simulink model "final_quadruped_060722_alphaobjfun"  (R2021a)
settings: Solver=ode15s  StartTime=0.0  StopTime=10  FixedStep=1e-3  RelTol=1e-5  EnableMultiTasking=on
values from neighbouring files (symbols this model uses):
  foot_x = 8    [bipedparameters.m]    (also in fcn.m; finalrobotParameters.m; finalrobotParameters_110522.m; finalrobotParameters_140522.m)
  foot_y = 6    [bipedparameters.m]    (also in fcn.m; finalrobotParameters.m; finalrobotParameters_110522.m; finalrobotParameters_140522.m)
  foot_z = 1    [bipedparameters.m]    (also in fcn.m; finalrobotParameters.m; finalrobotParameters_110522.m; finalrobotParameters_140522.m)
  height_plane = 0.025    [bipedparameters.m]    (also in finalrobotParameters.m; finalrobotParameters_110522.m; finalrobotParameters_140522.m; finalrobotParameters_240522.m)
  kd_ankle = 1000    [bipedparameters.m]    (also in finalrobotParameters_240522.m)
  kd_hip = 1000    [bipedparameters.m]    (also in finalrobotParameters_240522.m)
  kd_knee = 1000    [bipedparameters.m]    (also in finalrobotParameters_240522.m)
  ki_ankle = 1000    [bipedparameters.m]    (also in finalrobotParameters_240522.m)
  ki_hip = 1000    [bipedparameters.m]    (also in finalrobotParameters_240522.m)
  ki_knee = 2000    [bipedparameters.m]    (also in finalrobotParameters_240522.m)
  kp_ankle = 1000    [bipedparameters.m]    (also in finalrobotParameters_240522.m)
  kp_hip = 1000    [bipedparameters.m]    (also in finalrobotParameters_240522.m)
  kp_knee = 2000    [bipedparameters.m]    (also in finalrobotParameters_240522.m)
  lower_leg_length = 10    [bipedparameters.m]    (also in fcn.m; finalrobotParameters.m; finalrobotParameters_110522.m; finalrobotParameters_140522.m)
  plane_x = 25    [bipedparameters.m]    (also in finalrobotParameters.m; finalrobotParameters_110522.m; finalrobotParameters_140522.m; finalrobotParameters_240522.m)
  plane_y = 3    [bipedparameters.m]    (also in finalrobotParameters.m; finalrobotParameters_110522.m; finalrobotParameters_140522.m; finalrobotParameters_240522.m)
  torso_offset_x = -0.5    [bipedparameters.m]    (also in finalrobotParameters.m = 10; finalrobotParameters_110522.m = 10; finalrobotParameters_140522.m = 10; finalrobotParameters_240522.m = 10)
  torso_offset_z = -2    [bipedparameters.m]    (also in finalrobotParameters.m; finalrobotParameters_110522.m; finalrobotParameters_140522.m; finalrobotParameters_240522.m)
  torso_x = 5    [bipedparameters.m]    (also in fcn.m = 25; finalrobotParameters.m = 25; finalrobotParameters_110522.m = 25; finalrobotParameters_140522.m = 25)
  torso_y = 10    [bipedparameters.m]    (also in fcn.m = 16; finalrobotParameters.m = 16; finalrobotParameters_110522.m = 16; finalrobotParameters_140522.m = 16)
  torso_z = 8    [bipedparameters.m]    (also in fcn.m = 10; finalrobotParameters.m = 10; finalrobotParameters_110522.m = 10; finalrobotParameters_140522.m = 10)
  upper_leg_length = 10    [bipedparameters.m]    (also in fcn.m; finalrobotParameters.m; finalrobotParameters_110522.m; finalrobotParameters_140522.m)
undefined symbols (not defined in the file or in its folder): sigbuilder_block, X, Y, Z
libraries: nesl_utility x288, sm_lib x71, pid_lib x20, Contact_Forces_Lib x16, fl_lib x3
(part 6 of 9)

== system final_quadruped_060722_alphaobjfun/Model/Left Leg Front /Ankle  ==
  note: accelerationRFankle
  tddLF_ankle : Inport
  t2ddankle : Inport  Port=2
  Ankle : sm_lib/Joints/Revolute Joint  JointMode=Normal  SenseConstraintForce=off  SenseConstraintForceX=off  SenseConstraintForceY=off  SenseConstraintForceZ=off  SenseConstraintTorque=off  SenseConstraintTorqueX=off  SenseConstraintTorqueY=off  SenseConstraintTorqueZ=off  SenseTotalForce=off  SenseTotalForceX=off  SenseTotalForceY=off  SenseTotalForceZ=off  SenseTotalTorque=off  SenseTotalTorqueX=off  SenseTotalTorqueY=off  SenseTotalTorqueZ=off  CompositeWrenchDir=FollowerOnBase  CompositeWrenchFrame=BaseFrame  EquilibriumPosition=0  EquilibriumPositionUnits=deg  SpringStiffness=0  SpringStiffnessUnits=N*m/deg  DampingCoefficient=0  DampingCoefficientUnits=N*m/(deg/s)  TorqueActuationMode=InputTorque  MotionActuationMode=ComputedMotion  SensePosition=on  SenseVelocity=on  SenseAcceleration=on  SenseTorqueForce=off  SenseLowerLimitTorqueForce=off  SenseUpperLimitTorqueForce=off  LowerLimitSpecify=off  LowerLimitBound=-90  LowerLimitBoundUnits=deg  LowerLimitStiffness=1e4  LowerLimitStiffnessUnits=N*m/deg  LowerLimitDamping=10  LowerLimitDampingUnits=N*m/(deg/s)  LowerLimitTransitionRegionWidth=0.1  LowerLimitTransitionRegionWidthUnits=deg  UpperLimitSpecify=off  UpperLimitBound=90  UpperLimitBoundUnits=deg  UpperLimitStiffness=1e4  UpperLimitStiffnessUnits=N*m/deg  UpperLimitDamping=10  UpperLimitDampingUnits=N*m/(deg/s)  UpperLimitTransitionRegionWidth=0.1  UpperLimitTransitionRegionWidthUnits=deg  PositionTargetSpecify=on  PositionTargetPriority=Low  PositionTargetValue=-10  PositionTargetValueUnits=deg  VelocityTargetSpecify=on  VelocityTargetPriority=Low  VelocityTargetValue=1  VelocityTargetValueUnits=deg/s
  Bus Creator : BusCreator  Inputs=3
  PID Controller : pid_lib/PID Controller  Controller=PID  Form=Parallel  TimeDomain=Continuous-time  UseExternalTs=off  SampleTime=-1  IntegratorMethod=Forward Euler  FilterMethod=Forward Euler  ControllerParametersSource=internal  P=kp_ankle  I=ki_ankle  D=kd_ankle  UseFilter=on  N=100  TunerSelectOption=Transfer Function Based (PID Tuner App)  InitialConditionSource=internal  InitialConditionForIntegrator=0  InitialConditionForFilter=0  DifferentiatorICPrevScaledInput=0  ExternalReset=none  TrackingMode=off  Kt=1  LimitOutput=off  SatLimitsSource=internal  UpperSaturationLimit=inf  LowerSaturationLimit=-inf  LinearizeAsGain=on  AntiWindupMode=none  Kb=1  POutMin=[]  POutMax=[]  IOutMin=[]  IOutMax=[]  DOutMin=[]  DOutMax=[]  NOutMin=[]  NOutMax=[]  SumOutMin=[]  SumOutMax=[]  SaturationOutMin=[]  SaturationOutMax=[]  PParamMin=[]  PParamMax=[]  IParamMin=[]  IParamMax=[]  DParamMin=[]  DParamMax=[]  NParamMin=[]  NParamMax=[]  KbParamMin=[]  KbParamMax=[]  KtParamMin=[]  KtParamMax=[]  KbOutMin=[]  KbOutMax=[]  KtOutMin=[]  KtOutMax=[]  IntegratorOutMin=[]  IntegratorOutMax=[]  FilterOutMin=[]  FilterOutMax=[]  SumI1OutMin=[]  SumI1OutMax=[]  SumI2OutMin=[]  SumI2OutMax=[]  SumI3OutMin=[]  SumI3OutMax=[]  SumI4OutMin=[]  SumI4OutMax=[]  SumDOutMin=[]  SumDOutMax=[]  DifferentiatorOutMin=[]  DifferentiatorOutMax=[]  FilterDiffOutCoefMin=[]  FilterDiffOutCoefMax=[]  ReciprocalOutMin=[]  ReciprocalOutMax=[]  SumDenOutMin=[]  SumDenOutMax=[]  SumNumOutMin=[]  SumNumOutMax=[]  DivideOutMin=[]  DivideOutMax=[]  UdiffTsProdOutMin=[]  UdiffTsProdOutMax=[]  NTsProdOutMin=[]  NTsProdOutMax=[]  UintegralTsProdOutMin=[]  UintegralTsProdOutMax=[]  UngainTsProdOutMin=[]  UngainTsProdOutMax=[]  IntegratorContinuousStateAttributes=''  IntegratorStateMustResolveToSignalObject=off  IntegratorRTWStateStorageClass=Auto  FilterContinuousStateAttributes=''  FilterStateMustResolveToSignalObject=off  FilterRTWStateStorageClass=Auto  ParallelPVariant=InternalParameters  IdealPVariant=Disabled  IVariant=InternalParameters  DVariant=InternalParameters  IntegratorVariant=Continuous  SatVariant=Disabled  AWVariant=Passthrough  PCopyVariant=Disabled  TRVariant=Disabled  FdbkBlocksVariant=Forward  IdealPFdbkVariant=Disabled  SatFdbkVariant=Disabled  DerivativeFilterVariant=ContFilter  NVariant=InternalParameters  NCopyVariant=Disabled  FilterICVariant=InternalICsFilter  IntegratorICVariant=InternalICs  ExternalResetVariant=Disabled  TRSumVariant=Passthrough  SumFdbkVariant=Disabled  SumVariant=Sum_PID  TsampFilterVariant=InternalTs  TsampNgainVariant=Passthrough  TsampIntegralVariant=Passthrough  ExternalSaturationOutDataTypeStr=Inherit: Same as second input
  PS-Simulink Converter : nesl_utility/PS-Simulink Converter  PhysicalDomain=network_engine_domain  SubClassName=ps_output  LeftPortType=input  RightPortType=output  PseudoPeriodic=off  Frequencies=[]  Unit=1  AffineConversion=off
      settings: SourceProductBaseCode=PW,SS
  PS-Simulink Converter1 : nesl_utility/PS-Simulink Converter  PhysicalDomain=network_engine_domain  SubClassName=ps_output  LeftPortType=input  RightPortType=output  PseudoPeriodic=off  Frequencies=[]  Unit=1  AffineConversion=off
      settings: SourceProductBaseCode=PW,SS
  PS-Simulink Converter2 : nesl_utility/PS-Simulink Converter  PhysicalDomain=network_engine_domain  SubClassName=ps_output  LeftPortType=input  RightPortType=output  PseudoPeriodic=off  Frequencies=[]  Unit=inherit  AffineConversion=off
      settings: SourceProductBaseCode=PW,SS
  PS-Simulink Converter3 : nesl_utility/PS-Simulink Converter  PhysicalDomain=network_engine_domain  SubClassName=ps_output  LeftPortType=input  RightPortType=output  PseudoPeriodic=off  Frequencies=[]  Unit=inherit  AffineConversion=off
      settings: SourceProductBaseCode=PW,SS
  PS-Simulink Converter4 : nesl_utility/PS-Simulink Converter  PhysicalDomain=network_engine_domain  SubClassName=ps_output  LeftPortType=input  RightPortType=output  PseudoPeriodic=off  Frequencies=[]  Unit=inherit  AffineConversion=off
      settings: SourceProductBaseCode=PW,SS
  Scope : Scope
  Scope1 : Scope
  Scope2 : Scope
  Simulink-PS Converter : nesl_utility/Simulink-PS Converter  PhysicalDomain=network_engine_domain  SubClassName=ps_input  LeftPortType=input  RightPortType=output  PseudoPeriodic=off  Frequencies=[]  NoiseDistribution=none  NoiseParameters=[]  Unit=1  AffineConversion=off  FilteringAndDerivatives=provide  SimscapeFilterOrder=1  InputFilterTimeConstant=0.001  UdotUserProvided=0
      settings: SourceProductBaseCode=PW,SS
  Sum : Sum  Inputs=|+-
  B : PMIOPort  Side=Left
  F : PMIOPort  Port=2  Side=Right
  meas : Outport  VectorParamsAs1DForOutWhenUnconnected=off
  Outport : Outport  Port=2
  Outport1 : Outport  Port=3
  Outport2 : Outport  Port=4
  wires:
  PS-Simulink Converter1/1 -> Bus Creator/1  "angleRFankle"
  PS-Simulink Converter/1 -> Outport1/1, Bus Creator/2  "speedRFankle"
  PID Controller/1 -> Scope1/1, Simulink-PS Converter/1, Bus Creator/3  "torqueRFankle"
  Bus Creator/1 -> meas/1
  Sum/1 -> PID Controller/1, Scope/1
  PS-Simulink Converter2/1 -> Outport/1
  PS-Simulink Converter3/1 -> Outport2/1
  PS-Simulink Converter4/1 -> Sum/2
  tddLF_ankle/1 -> Sum/1
  t2ddankle/1 -> Scope2/1
  connections:
  F/RConn1 -- Ankle/RConn1
  Ankle/LConn1 -- B/RConn1
  PS-Simulink Converter1/LConn1 -- Ankle/RConn2 -- PS-Simulink Converter2/LConn1
  Ankle/RConn3 -- PS-Simulink Converter4/LConn1 -- PS-Simulink Converter/LConn1
  Simulink-PS Converter/RConn1 -- Ankle/LConn2
  Ankle/RConn4 -- PS-Simulink Converter3/LConn1

== system final_quadruped_060722_alphaobjfun/Model/Left Leg Front /Contact Forces  ==
  In1 : Inport
  In2 : Inport  Port=2
  In3 : Inport  Port=3
  Qd3g : Inport  Port=4
  In4 : Inport  Port=5
  pfLF : Inport  Port=6
  Add : Sum  Inputs=++++
  Add1 : Sum  Inputs=++++
  Bus Selector{,1..3} (4 alike) : BusSelector  OutputSignals=Normal Force,Friction Force
  MATLAB Function : MATLAB Function  TreatAsAtomicUnit=on
  MATLAB Function1 : MATLAB Function  TreatAsAtomicUnit=on
  Math Function : Math  Operator=square  SignedPower=on  SaturateOnIntegerOverflow=on
  Scope : Scope
  Scope1 : Scope
  Sqrt : Sqrt  SaturateOnIntegerOverflow=on
  Sum of Elements : Sum  Inputs=+
  Outport : Outport
  Outport1 : Outport  Port=2
  pNLF : Outport  Port=3
  p1 : Outport  Port=4
  p2 : Outport  Port=5
  p3 : Outport  Port=6
  p4 : Outport  Port=7
  n1 : Outport  Port=8
  n2 : Outport  Port=9
  n3 : Outport  Port=10
  n4 : Outport  Port=11
  wires:
  Sqrt/1 -> ?
  Add/1 -> ?
  Sum of Elements/1 -> Sqrt/1
  Bus Selector1/2 -> Add1/2, MATLAB Function/6(f2)  "<Friction Force>"
  Bus Selector2/1 -> n3/1, MATLAB Function1/3(n3), MATLAB Function/4(n3), Add/3  "<Normal Force>"
  Bus Selector3/2 -> Scope1/1, MATLAB Function/8(f4), Add1/4  "<Friction Force>"
  Bus Selector3/1 -> Add/4, MATLAB Function/3(n4), n4/1, MATLAB Function1/4(n4)  "<Normal Force>"
  Bus Selector/1 -> Add/1, Scope/1, n1/1, MATLAB Function1/1(n1), MATLAB Function/1(n1)  "<Normal Force>"
  Bus Selector/2 -> MATLAB Function/5(f1), Add1/1  "<Friction Force>"
  Bus Selector1/1 -> Add/2, n2/1, MATLAB Function1/2(n2), MATLAB Function/2(n2)  "<Normal Force>"
  In3/1 -> Bus Selector2/1
  Add1/1 -> Math Function/1
  Math Function/1 -> Sum of Elements/1
  In2/1 -> Bus Selector1/1
  Bus Selector2/2 -> MATLAB Function/7(f3), Add1/3  "<Friction Force>"
  In1/1 -> Bus Selector/1
  In4/1 -> Bus Selector3/1
  MATLAB Function/1(NRF) -> Outport/1
  MATLAB Function/2(FRF) -> Outport1/1
  Qd3g/1 -> MATLAB Function1/5(Qd5g), MATLAB Function/9(Qd3g)
  pfLF/1 -> MATLAB Function1/6(pfLF)
  MATLAB Function1/1(pNLF) -> pNLF/1
  MATLAB Function1/2(p1) -> p1/1
  MATLAB Function1/3(p2) -> p2/1
  MATLAB Function1/4(p3) -> p3/1
  MATLAB Function1/5(p4) -> p4/1

== system final_quadruped_060722_alphaobjfun/Model/Left Leg Front /Hip ==
  note: accelerationRFhip
  t2ddhip : Inport
  tddLF_hip : Inport  Port=2
  Gimbal Joint : sm_lib/Joints/Gimbal Joint  JointMode=Normal  SenseConstraintForce=off  SenseConstraintForceX=off  SenseConstraintForceY=off  SenseConstraintForceZ=off  SenseConstraintTorque=off  SenseConstraintTorqueX=off  SenseConstraintTorqueY=off  SenseConstraintTorqueZ=off  SenseTotalForce=off  SenseTotalForceX=off  SenseTotalForceY=off  SenseTotalForceZ=off  SenseTotalTorque=off  SenseTotalTorqueX=off  SenseTotalTorqueY=off  SenseTotalTorqueZ=off  CompositeWrenchDir=FollowerOnBase  CompositeWrenchFrame=BaseFrame  RxEquilibriumPosition=0  RxEquilibriumPositionUnits=deg  RxSpringStiffness=0  RxSpringStiffnessUnits=N*m/deg  RxDampingCoefficient=0  RxDampingCoefficientUnits=N*m/(deg/s)  RxTorqueActuationMode=InputTorque  RxMotionActuationMode=ComputedMotion  RxSensePosition=on  RxSenseVelocity=on  RxSenseAcceleration=on  RxSenseTorqueForce=off  RxSenseLowerLimitTorqueForce=off  RxSenseUpperLimitTorqueForce=off  RxLowerLimitSpecify=off  RxLowerLimitBound=-90  RxLowerLimitBoundUnits=deg  RxLowerLimitStiffness=1e4  RxLowerLimitStiffnessUnits=N*m/deg  RxLowerLimitDamping=10  RxLowerLimitDampingUnits=N*m/(deg/s)  RxLowerLimitTransitionRegionWidth=0.1  RxLowerLimitTransitionRegionWidthUnits=deg  RxUpperLimitSpecify=off  RxUpperLimitBound=90  RxUpperLimitBoundUnits=deg  RxUpperLimitStiffness=1e4  RxUpperLimitStiffnessUnits=N*m/deg  RxUpperLimitDamping=10  RxUpperLimitDampingUnits=N*m/(deg/s)  RxUpperLimitTransitionRegionWidth=0.1  RxUpperLimitTransitionRegionWidthUnits=deg  RxPositionTargetSpecify=off  RxPositionTargetPriority=High  RxPositionTargetValue=0  RxPositionTargetValueUnits=deg  RxVelocityTargetSpecify=off  RxVelocityTargetPriority=High  RxVelocityTargetValue=0  RxVelocityTargetValueUnits=deg/s  RyEquilibriumPosition=0  RyEquilibriumPositionUnits=deg  RySpringStiffness=0  RySpringStiffnessUnits=N*m/deg  RyDampingCoefficient=0  RyDampingCoefficientUnits=N*m/(deg/s)  RyTorqueActuationMode=InputTorque  RyMotionActuationMode=ComputedMotion  RySensePosition=on  RySenseVelocity=on  RySenseAcceleration=on  RySenseTorqueForce=off  RySenseLowerLimitTorqueForce=off  RySenseUpperLimitTorqueForce=off  RyLowerLimitSpecify=off  RyLowerLimitBound=-90  RyLowerLimitBoundUnits=deg  RyLowerLimitStiffness=1e4  RyLowerLimitStiffnessUnits=N*m/deg  RyLowerLimitDamping=10  RyLowerLimitDampingUnits=N*m/(deg/s)  RyLowerLimitTransitionRegionWidth=0.1  RyLowerLimitTransitionRegionWidthUnits=deg  RyUpperLimitSpecify=off  RyUpperLimitBound=90  RyUpperLimitBoundUnits=deg  RyUpperLimitStiffness=1e4  RyUpperLimitStiffnessUnits=N*m/deg  RyUpperLimitDamping=10  RyUpperLimitDampingUnits=N*m/(deg/s)  RyUpperLimitTransitionRegionWidth=0.1  RyUpperLimitTransitionRegionWidthUnits=deg  RyPositionTargetSpecify=off  RyPositionTargetPriority=High  RyPositionTargetValue=0  RyPositionTargetValueUnits=deg  RyVelocityTargetSpecify=off  RyVelocityTargetPriority=High  RyVelocityTargetValue=0  RyVelocityTargetValueUnits=deg/s  RzEquilibriumPosition=0  RzEquilibriumPositionUnits=deg  RzSpringStiffness=0  RzSpringStiffnessUnits=N*m/deg  RzDampingCoefficient=0  RzDampingCoefficientUnits=N*m/(deg/s)  RzTorqueActuationMode=InputTorque  RzMotionActuationMode=ComputedMotion  RzSensePosition=on  RzSenseVelocity=on  RzSenseAcceleration=on  RzSenseTorqueForce=off  RzSenseLowerLimitTorqueForce=off  RzSenseUpperLimitTorqueForce=off  RzLowerLimitSpecify=off  RzLowerLimitBound=-90  RzLowerLimitBoundUnits=deg  RzLowerLimitStiffness=1e4  RzLowerLimitStiffnessUnits=N*m/deg  RzLowerLimitDamping=10  RzLowerLimitDampingUnits=N*m/(deg/s)  RzLowerLimitTransitionRegionWidth=0.1  RzLowerLimitTransitionRegionWidthUnits=deg  RzUpperLimitSpecify=off  RzUpperLimitBound=90  RzUpperLimitBoundUnits=deg  RzUpperLimitStiffness=1e4  RzUpperLimitStiffnessUnits=N*m/deg  RzUpperLimitDamping=10  RzUpperLimitDampingUnits=N*m/(deg/s)  RzUpperLimitTransitionRegionWidth=0.1  RzUpperLimitTransitionRegionWidthUnits=deg  RzPositionTargetSpecify=on  RzPositionTargetPriority=Low  RzPositionTargetValue=-10  RzPositionTargetValueUnits=deg  RzVelocityTargetSpecify=on  RzVelocityTargetPriority=Low  RzVelocityTargetValue=1  RzVelocityTargetValueUnits=deg/s
  MATLAB Function : MATLAB Function  TreatAsAtomicUnit=on
  MATLAB Function1 : MATLAB Function  TreatAsAtomicUnit=on
  MATLAB Function2 : MATLAB Function  TreatAsAtomicUnit=on
  MATLAB Function3 : MATLAB Function  TreatAsAtomicUnit=on
  PID Controller : pid_lib/PID Controller  Controller=PID  Form=Parallel  TimeDomain=Continuous-time  UseExternalTs=off  SampleTime=-1  IntegratorMethod=Forward Euler  FilterMethod=Forward Euler  ControllerParametersSource=internal  P=kp_hip  I=ki_hip  D=kd_hip  UseFilter=on  N=100  TunerSelectOption=Transfer Function Based (PID Tuner App)  InitialConditionSource=internal  InitialConditionForIntegrator=0  InitialConditionForFilter=0  DifferentiatorICPrevScaledInput=0  ExternalReset=none  TrackingMode=off  Kt=1  LimitOutput=off  SatLimitsSource=internal  UpperSaturationLimit=inf  LowerSaturationLimit=-inf  LinearizeAsGain=on  AntiWindupMode=none  Kb=1  POutMin=[]  POutMax=[]  IOutMin=[]  IOutMax=[]  DOutMin=[]  DOutMax=[]  NOutMin=[]  NOutMax=[]  SumOutMin=[]  SumOutMax=[]  SaturationOutMin=[]  SaturationOutMax=[]  PParamMin=[]  PParamMax=[]  IParamMin=[]  IParamMax=[]  DParamMin=[]  DParamMax=[]  NParamMin=[]  NParamMax=[]  KbParamMin=[]  KbParamMax=[]  KtParamMin=[]  KtParamMax=[]  KbOutMin=[]  KbOutMax=[]  KtOutMin=[]  KtOutMax=[]  IntegratorOutMin=[]  IntegratorOutMax=[]  FilterOutMin=[]  FilterOutMax=[]  SumI1OutMin=[]  SumI1OutMax=[]  SumI2OutMin=[]  SumI2OutMax=[]  SumI3OutMin=[]  SumI3OutMax=[]  SumI4OutMin=[]  SumI4OutMax=[]  SumDOutMin=[]  SumDOutMax=[]  DifferentiatorOutMin=[]  DifferentiatorOutMax=[]  FilterDiffOutCoefMin=[]  FilterDiffOutCoefMax=[]  ReciprocalOutMin=[]  ReciprocalOutMax=[]  SumDenOutMin=[]  SumDenOutMax=[]  SumNumOutMin=[]  SumNumOutMax=[]  DivideOutMin=[]  DivideOutMax=[]  UdiffTsProdOutMin=[]  UdiffTsProdOutMax=[]  NTsProdOutMin=[]  NTsProdOutMax=[]  UintegralTsProdOutMin=[]  UintegralTsProdOutMax=[]  UngainTsProdOutMin=[]  UngainTsProdOutMax=[]  IntegratorContinuousStateAttributes=''  IntegratorStateMustResolveToSignalObject=off  IntegratorRTWStateStorageClass=Auto  FilterContinuousStateAttributes=''  FilterStateMustResolveToSignalObject=off  FilterRTWStateStorageClass=Auto  ParallelPVariant=InternalParameters  IdealPVariant=Disabled  IVariant=InternalParameters  DVariant=InternalParameters  IntegratorVariant=Continuous  SatVariant=Disabled  AWVariant=Passthrough  PCopyVariant=Disabled  TRVariant=Disabled  FdbkBlocksVariant=Forward  IdealPFdbkVariant=Disabled  SatFdbkVariant=Disabled  DerivativeFilterVariant=ContFilter  NVariant=InternalParameters  NCopyVariant=Disabled  FilterICVariant=InternalICsFilter  IntegratorICVariant=InternalICs  ExternalResetVariant=Disabled  TRSumVariant=Passthrough  SumFdbkVariant=Disabled  SumVariant=Sum_PID  TsampFilterVariant=InternalTs  TsampNgainVariant=Passthrough  TsampIntegralVariant=Passthrough  ExternalSaturationOutDataTypeStr=Inherit: Same as second input
  PID Controller1 : pid_lib/PID Controller  Controller=PID  Form=Parallel  TimeDomain=Continuous-time  UseExternalTs=off  SampleTime=-1  IntegratorMethod=Forward Euler  FilterMethod=Forward Euler  ControllerParametersSource=internal  P=kp_hip  I=ki_hip  D=kd_hip  UseFilter=on  N=100  TunerSelectOption=Transfer Function Based (PID Tuner App)  InitialConditionSource=internal  InitialConditionForIntegrator=0  InitialConditionForFilter=0  DifferentiatorICPrevScaledInput=0  ExternalReset=none  TrackingMode=off  Kt=1  LimitOutput=off  SatLimitsSource=internal  UpperSaturationLimit=inf  LowerSaturationLimit=-inf  LinearizeAsGain=on  AntiWindupMode=none  Kb=1  POutMin=[]  POutMax=[]  IOutMin=[]  IOutMax=[]  DOutMin=[]  DOutMax=[]  NOutMin=[]  NOutMax=[]  SumOutMin=[]  SumOutMax=[]  SaturationOutMin=[]  SaturationOutMax=[]  PParamMin=[]  PParamMax=[]  IParamMin=[]  IParamMax=[]  DParamMin=[]  DParamMax=[]  NParamMin=[]  NParamMax=[]  KbParamMin=[]  KbParamMax=[]  KtParamMin=[]  KtParamMax=[]  KbOutMin=[]  KbOutMax=[]  KtOutMin=[]  KtOutMax=[]  IntegratorOutMin=[]  IntegratorOutMax=[]  FilterOutMin=[]  FilterOutMax=[]  SumI1OutMin=[]  SumI1OutMax=[]  SumI2OutMin=[]  SumI2OutMax=[]  SumI3OutMin=[]  SumI3OutMax=[]  SumI4OutMin=[]  SumI4OutMax=[]  SumDOutMin=[]  SumDOutMax=[]  DifferentiatorOutMin=[]  DifferentiatorOutMax=[]  FilterDiffOutCoefMin=[]  FilterDiffOutCoefMax=[]  ReciprocalOutMin=[]  ReciprocalOutMax=[]  SumDenOutMin=[]  SumDenOutMax=[]  SumNumOutMin=[]  SumNumOutMax=[]  DivideOutMin=[]  DivideOutMax=[]  UdiffTsProdOutMin=[]  UdiffTsProdOutMax=[]  NTsProdOutMin=[]  NTsProdOutMax=[]  UintegralTsProdOutMin=[]  UintegralTsProdOutMax=[]  UngainTsProdOutMin=[]  UngainTsProdOutMax=[]  IntegratorContinuousStateAttributes=''  IntegratorStateMustResolveToSignalObject=off  IntegratorRTWStateStorageClass=Auto  FilterContinuousStateAttributes=''  FilterStateMustResolveToSignalObject=off  FilterRTWStateStorageClass=Auto  ParallelPVariant=InternalParameters  IdealPVariant=Disabled  IVariant=InternalParameters  DVariant=InternalParameters  IntegratorVariant=Continuous  SatVariant=Disabled  AWVariant=Passthrough  PCopyVariant=Disabled  TRVariant=Disabled  FdbkBlocksVariant=Forward  IdealPFdbkVariant=Disabled  SatFdbkVariant=Disabled  DerivativeFilterVariant=ContFilter  NVariant=InternalParameters  NCopyVariant=Disabled  FilterICVariant=InternalICsFilter  IntegratorICVariant=InternalICs  ExternalResetVariant=Disabled  TRSumVariant=Passthrough  SumFdbkVariant=Disabled  SumVariant=Sum_PID  TsampFilterVariant=InternalTs  TsampNgainVariant=Passthrough  TsampIntegralVariant=Passthrough  ExternalSaturationOutDataTypeStr=Inherit: Same as second input
  PID Controller2 : pid_lib/PID Controller  Controller=PID  Form=Parallel  TimeDomain=Continuous-time  UseExternalTs=off  SampleTime=-1  IntegratorMethod=Forward Euler  FilterMethod=Forward Euler  ControllerParametersSource=internal  P=kp_hip  I=ki_hip  D=kd_hip  UseFilter=on  N=100  TunerSelectOption=Transfer Function Based (PID Tuner App)  InitialConditionSource=internal  InitialConditionForIntegrator=0  InitialConditionForFilter=0  DifferentiatorICPrevScaledInput=0  ExternalReset=none  TrackingMode=off  Kt=1  LimitOutput=off  SatLimitsSource=internal  UpperSaturationLimit=inf  LowerSaturationLimit=-inf  LinearizeAsGain=on  AntiWindupMode=none  Kb=1  POutMin=[]  POutMax=[]  IOutMin=[]  IOutMax=[]  DOutMin=[]  DOutMax=[]  NOutMin=[]  NOutMax=[]  SumOutMin=[]  SumOutMax=[]  SaturationOutMin=[]  SaturationOutMax=[]  PParamMin=[]  PParamMax=[]  IParamMin=[]  IParamMax=[]  DParamMin=[]  DParamMax=[]  NParamMin=[]  NParamMax=[]  KbParamMin=[]  KbParamMax=[]  KtParamMin=[]  KtParamMax=[]  KbOutMin=[]  KbOutMax=[]  KtOutMin=[]  KtOutMax=[]  IntegratorOutMin=[]  IntegratorOutMax=[]  FilterOutMin=[]  FilterOutMax=[]  SumI1OutMin=[]  SumI1OutMax=[]  SumI2OutMin=[]  SumI2OutMax=[]  SumI3OutMin=[]  SumI3OutMax=[]  SumI4OutMin=[]  SumI4OutMax=[]  SumDOutMin=[]  SumDOutMax=[]  DifferentiatorOutMin=[]  DifferentiatorOutMax=[]  FilterDiffOutCoefMin=[]  FilterDiffOutCoefMax=[]  ReciprocalOutMin=[]  ReciprocalOutMax=[]  SumDenOutMin=[]  SumDenOutMax=[]  SumNumOutMin=[]  SumNumOutMax=[]  DivideOutMin=[]  DivideOutMax=[]  UdiffTsProdOutMin=[]  UdiffTsProdOutMax=[]  NTsProdOutMin=[]  NTsProdOutMax=[]  UintegralTsProdOutMin=[]  UintegralTsProdOutMax=[]  UngainTsProdOutMin=[]  UngainTsProdOutMax=[]  IntegratorContinuousStateAttributes=''  IntegratorStateMustResolveToSignalObject=off  IntegratorRTWStateStorageClass=Auto  FilterContinuousStateAttributes=''  FilterStateMustResolveToSignalObject=off  FilterRTWStateStorageClass=Auto  ParallelPVariant=InternalParameters  IdealPVariant=Disabled  IVariant=InternalParameters  DVariant=InternalParameters  IntegratorVariant=Continuous  SatVariant=Disabled  AWVariant=Passthrough  PCopyVariant=Disabled  TRVariant=Disabled  FdbkBlocksVariant=Forward  IdealPFdbkVariant=Disabled  SatFdbkVariant=Disabled  DerivativeFilterVariant=ContFilter  NVariant=InternalParameters  NCopyVariant=Disabled  FilterICVariant=InternalICsFilter  IntegratorICVariant=InternalICs  ExternalResetVariant=Disabled  TRSumVariant=Passthrough  SumFdbkVariant=Disabled  SumVariant=Sum_PID  TsampFilterVariant=InternalTs  TsampNgainVariant=Passthrough  TsampIntegralVariant=Passthrough  ExternalSaturationOutDataTypeStr=Inherit: Same as second input
  PS-Simulink Converter{,2..11} (11 alike) : nesl_utility/PS-Simulink Converter  PhysicalDomain=network_engine_domain  SubClassName=ps_output  LeftPortType=input  RightPortType=output  PseudoPeriodic=off  Frequencies=[]  Unit=inherit  AffineConversion=off
      settings: SourceProductBaseCode=PW,SS
  PS-Simulink Converter1 : nesl_utility/PS-Simulink Converter  PhysicalDomain=network_engine_domain  SubClassName=ps_output  LeftPortType=input  RightPortType=output  PseudoPeriodic=off  Frequencies=[]  Unit=1  AffineConversion=off
      settings: SourceProductBaseCode=PW,SS
  Scope{,1..6} (7 alike) : Scope
  Simulink-PS Converter : nesl_utility/Simulink-PS Converter  PhysicalDomain=network_engine_domain  SubClassName=ps_input  LeftPortType=input  RightPortType=output  PseudoPeriodic=off  Frequencies=[]  NoiseDistribution=none  NoiseParameters=[]  Unit=1  AffineConversion=off  FilteringAndDerivatives=provide  SimscapeFilterOrder=1  InputFilterTimeConstant=0.001  UdotUserProvided=0
      settings: SourceProductBaseCode=PW,SS
  Simulink-PS Converter1 : nesl_utility/Simulink-PS Converter  PhysicalDomain=network_engine_domain  SubClassName=ps_input  LeftPortType=input  RightPortType=output  PseudoPeriodic=off  Frequencies=[]  NoiseDistribution=none  NoiseParameters=[]  Unit=1  AffineConversion=off  FilteringAndDerivatives=provide  SimscapeFilterOrder=1  InputFilterTimeConstant=0.001  UdotUserProvided=0
      settings: SourceProductBaseCode=PW,SS
  Simulink-PS Converter2 : nesl_utility/Simulink-PS Converter  PhysicalDomain=network_engine_domain  SubClassName=ps_input  LeftPortType=input  RightPortType=output  PseudoPeriodic=off  Frequencies=[]  NoiseDistribution=none  NoiseParameters=[]  Unit=1  AffineConversion=off  FilteringAndDerivatives=provide  SimscapeFilterOrder=1  InputFilterTimeConstant=0.001  UdotUserProvided=0
      settings: SourceProductBaseCode=PW,SS
  Sum : Sum  Inputs=|+-
  Sum1 : Sum  Inputs=|+-
  Sum2 : Sum  Inputs=|+-
  Conn1 : PMIOPort  Side=Left
  Conn2 : PMIOPort  Port=2  Side=Right
  qx : PMIOPort  Port=3  Side=Right
  qy : PMIOPort  Port=4  Side=Right
  qz : PMIOPort  Port=5  Side=Right
  Outport2 : Outport
  Outport1 : Outport  Port=2
  Outport : Outport  Port=3
  wires:
  PS-Simulink Converter1/1 -> Sum/2  "speedRFhip"
  Sum/1 -> PID Controller/1, Scope/1
  PID Controller/1 -> Scope1/1, Simulink-PS Converter/1  "torqueRFhip"
  MATLAB Function1/1(hip) -> Outport2/1
  t2ddhip/1 -> Scope2/1
  PS-Simulink Converter/1 -> MATLAB Function/1(qx)
  PS-Simulink Converter4/1 -> MATLAB Function/2(qy)
  PS-Simulink Converter5/1 -> MATLAB Function/3(qz)
  MATLAB Function/1(hip) -> Outport1/1
  PS-Simulink Converter6/1 -> MATLAB Function1/1(wx)
  PS-Simulink Converter7/1 -> MATLAB Function1/2(wy)
  PS-Simulink Converter8/1 -> MATLAB Function1/3(wz)
  tddLF_hip/1 -> MATLAB Function2/1(tddRF)
  PID Controller1/1 -> Simulink-PS Converter1/1, Scope4/1  "torqueRFhip"
  Sum1/1 -> PID Controller1/1, Scope3/1
  MATLAB Function2/1(tddRFx) -> Sum1/1
  PS-Simulink Converter2/1 -> Sum1/2
  MATLAB Function2/3(tddRFz) -> Sum/1
  PID Controller2/1 -> Simulink-PS Converter2/1, Scope6/1  "torqueRFhip"
  Sum2/1 -> PID Controller2/1, Scope5/1
  MATLAB Function2/2(tddRFy) -> Sum2/1
  PS-Simulink Converter9/1 -> Sum2/2
  PS-Simulink Converter10/1 -> MATLAB Function3/1(bx)
  PS-Simulink Converter3/1 -> MATLAB Function3/3(bz)
  PS-Simulink Converter11/1 -> MATLAB Function3/2(by)
  MATLAB Function3/1(hip) -> Outport/1
  connections:
  Conn2/RConn1 -- Gimbal Joint/RConn1
  Conn1/RConn1 -- Gimbal Joint/LConn1
  Gimbal Joint/RConn2 -- qx/RConn1 -- PS-Simulink Converter/LConn1
  PS-Simulink Converter4/LConn1 -- Gimbal Joint/RConn5 -- qy/RConn1
  PS-Simulink Converter5/LConn1 -- Gimbal Joint/RConn8 -- qz/RConn1
  Gimbal Joint/RConn3 -- PS-Simulink Converter2/LConn1 -- PS-Simulink Converter6/LConn1
  PS-Simulink Converter7/LConn1 -- Gimbal Joint/RConn6 -- PS-Simulink Converter9/LConn1
  PS-Simulink Converter8/LConn1 -- Gimbal Joint/RConn9 -- PS-Simulink Converter1/LConn1
  Simulink-PS Converter1/RConn1 -- Gimbal Joint/LConn2
  Simulink-PS Converter2/RConn1 -- Gimbal Joint/LConn3
  Simulink-PS Converter/RConn1 -- Gimbal Joint/LConn4
  Gimbal Joint/RConn4 -- PS-Simulink Converter10/LConn1
  Gimbal Joint/RConn7 -- PS-Simulink Converter11/LConn1
  Gimbal Joint/RConn10 -- PS-Simulink Converter3/LConn1

== system final_quadruped_060722_alphaobjfun/Model/Left Leg Front /Knee ==
  note: accelerationRFknee
  note: Meas for knee
  tddLF_knee : Inport
  t2ddknee : Inport  Port=2
  Bus Creator : BusCreator  Inputs=3
  Knee joint : sm_lib/Joints/Revolute Joint  JointMode=Normal  SenseConstraintForce=off  SenseConstraintForceX=off  SenseConstraintForceY=off  SenseConstraintForceZ=off  SenseConstraintTorque=off  SenseConstraintTorqueX=off  SenseConstraintTorqueY=off  SenseConstraintTorqueZ=off  SenseTotalForce=off  SenseTotalForceX=off  SenseTotalForceY=off  SenseTotalForceZ=off  SenseTotalTorque=off  SenseTotalTorqueX=off  SenseTotalTorqueY=off  SenseTotalTorqueZ=off  CompositeWrenchDir=FollowerOnBase  CompositeWrenchFrame=BaseFrame  EquilibriumPosition=0  EquilibriumPositionUnits=deg  SpringStiffness=0  SpringStiffnessUnits=N*m/deg  DampingCoefficient=0  DampingCoefficientUnits=N*m/(deg/s)  TorqueActuationMode=InputTorque  MotionActuationMode=ComputedMotion  SensePosition=on  SenseVelocity=on  SenseAcceleration=on  SenseTorqueForce=off  SenseLowerLimitTorqueForce=off  SenseUpperLimitTorqueForce=off  LowerLimitSpecify=on  LowerLimitBound=0  LowerLimitBoundUnits=deg  LowerLimitStiffness=1e4  LowerLimitStiffnessUnits=N*m/deg  LowerLimitDamping=10  LowerLimitDampingUnits=N*m/(deg/s)  LowerLimitTransitionRegionWidth=0.1  LowerLimitTransitionRegionWidthUnits=deg  UpperLimitSpecify=on  UpperLimitBound=20  UpperLimitBoundUnits=deg  UpperLimitStiffness=1e4  UpperLimitStiffnessUnits=N*m/deg  UpperLimitDamping=10  UpperLimitDampingUnits=N*m/(deg/s)  UpperLimitTransitionRegionWidth=0.1  UpperLimitTransitionRegionWidthUnits=deg  PositionTargetSpecify=on  PositionTargetPriority=Low  PositionTargetValue=20  PositionTargetValueUnits=deg  VelocityTargetSpecify=on  VelocityTargetPriority=Low  VelocityTargetValue=-2  VelocityTargetValueUnits=deg/s
  PID Controller : pid_lib/PID Controller  Controller=PID  Form=Parallel  TimeDomain=Continuous-time  UseExternalTs=off  SampleTime=-1  IntegratorMethod=Forward Euler  FilterMethod=Forward Euler  ControllerParametersSource=internal  P=kp_knee  I=ki_knee  D=kd_knee  UseFilter=on  N=100  TunerSelectOption=Transfer Function Based (PID Tuner App)  InitialConditionSource=internal  InitialConditionForIntegrator=0  InitialConditionForFilter=0  DifferentiatorICPrevScaledInput=0  ExternalReset=none  TrackingMode=off  Kt=1  LimitOutput=off  SatLimitsSource=internal  UpperSaturationLimit=inf  LowerSaturationLimit=-inf  LinearizeAsGain=on  AntiWindupMode=none  Kb=1  POutMin=[]  POutMax=[]  IOutMin=[]  IOutMax=[]  DOutMin=[]  DOutMax=[]  NOutMin=[]  NOutMax=[]  SumOutMin=[]  SumOutMax=[]  SaturationOutMin=[]  SaturationOutMax=[]  PParamMin=[]  PParamMax=[]  IParamMin=[]  IParamMax=[]  DParamMin=[]  DParamMax=[]  NParamMin=[]  NParamMax=[]  KbParamMin=[]  KbParamMax=[]  KtParamMin=[]  KtParamMax=[]  KbOutMin=[]  KbOutMax=[]  KtOutMin=[]  KtOutMax=[]  IntegratorOutMin=[]  IntegratorOutMax=[]  FilterOutMin=[]  FilterOutMax=[]  SumI1OutMin=[]  SumI1OutMax=[]  SumI2OutMin=[]  SumI2OutMax=[]  SumI3OutMin=[]  SumI3OutMax=[]  SumI4OutMin=[]  SumI4OutMax=[]  SumDOutMin=[]  SumDOutMax=[]  DifferentiatorOutMin=[]  DifferentiatorOutMax=[]  FilterDiffOutCoefMin=[]  FilterDiffOutCoefMax=[]  ReciprocalOutMin=[]  ReciprocalOutMax=[]  SumDenOutMin=[]  SumDenOutMax=[]  SumNumOutMin=[]  SumNumOutMax=[]  DivideOutMin=[]  DivideOutMax=[]  UdiffTsProdOutMin=[]  UdiffTsProdOutMax=[]  NTsProdOutMin=[]  NTsProdOutMax=[]  UintegralTsProdOutMin=[]  UintegralTsProdOutMax=[]  UngainTsProdOutMin=[]  UngainTsProdOutMax=[]  IntegratorContinuousStateAttributes=''  IntegratorStateMustResolveToSignalObject=off  IntegratorRTWStateStorageClass=Auto  FilterContinuousStateAttributes=''  FilterStateMustResolveToSignalObject=off  FilterRTWStateStorageClass=Auto  ParallelPVariant=InternalParameters  IdealPVariant=Disabled  IVariant=InternalParameters  DVariant=InternalParameters  IntegratorVariant=Continuous  SatVariant=Disabled  AWVariant=Passthrough  PCopyVariant=Disabled  TRVariant=Disabled  FdbkBlocksVariant=Forward  IdealPFdbkVariant=Disabled  SatFdbkVariant=Disabled  DerivativeFilterVariant=ContFilter  NVariant=InternalParameters  NCopyVariant=Disabled  FilterICVariant=InternalICsFilter  IntegratorICVariant=InternalICs  ExternalResetVariant=Disabled  TRSumVariant=Passthrough  SumFdbkVariant=Disabled  SumVariant=Sum_PID  TsampFilterVariant=InternalTs  TsampNgainVariant=Passthrough  TsampIntegralVariant=Passthrough  ExternalSaturationOutDataTypeStr=Inherit: Same as second input
  PS-Simulink Converter : nesl_utility/PS-Simulink Converter  PhysicalDomain=network_engine_domain  SubClassName=ps_output  LeftPortType=input  RightPortType=output  PseudoPeriodic=off  Frequencies=[]  Unit=inherit  AffineConversion=off
      settings: SourceProductBaseCode=PW,SS
  PS-Simulink Converter1 : nesl_utility/PS-Simulink Converter  PhysicalDomain=network_engine_domain  SubClassName=ps_output  LeftPortType=input  RightPortType=output  PseudoPeriodic=off  Frequencies=[]  Unit=1  AffineConversion=off
      settings: SourceProductBaseCode=PW,SS
  PS-Simulink Converter2 : nesl_utility/PS-Simulink Converter  PhysicalDomain=network_engine_domain  SubClassName=ps_output  LeftPortType=input  RightPortType=output  PseudoPeriodic=off  Frequencies=[]  Unit=inherit  AffineConversion=off
      settings: SourceProductBaseCode=PW,SS
  PS-Simulink Converter3 : nesl_utility/PS-Simulink Converter  PhysicalDomain=network_engine_domain  SubClassName=ps_output  LeftPortType=input  RightPortType=output  PseudoPeriodic=off  Frequencies=[]  Unit=1  AffineConversion=off
      settings: SourceProductBaseCode=PW,SS
  Scope : Scope
  Scope1 : Scope
  Scope2 : Scope
  Simulink-PS Converter : nesl_utility/Simulink-PS Converter  PhysicalDomain=network_engine_domain  SubClassName=ps_input  LeftPortType=input  RightPortType=output  PseudoPeriodic=off  Frequencies=[]  NoiseDistribution=none  NoiseParameters=[]  Unit=1  AffineConversion=off  FilteringAndDerivatives=provide  SimscapeFilterOrder=1  InputFilterTimeConstant=0.001  UdotUserProvided=0
      settings: SourceProductBaseCode=PW,SS
  Sum : Sum  Inputs=|+-
  Conn1 : PMIOPort  Side=Left
  Conn2 : PMIOPort  Port=2  Side=Right
  q : PMIOPort  Port=3  Side=Left
  meas : Outport
  Outport : Outport  Port=2
  Outport2 : Outport  Port=3
  wires:
  Bus Creator/1 -> meas/1
  PS-Simulink Converter3/1 -> Bus Creator/1  "angleRFknee"
  PS-Simulink Converter1/1 -> Outport/1, Bus Creator/2  "speedRFknee"
  Sum/1 -> Scope1/1, PID Controller/1
  PID Controller/1 -> Bus Creator/3, Simulink-PS Converter/1, Scope/1  "torqueRFknee"
  PS-Simulink Converter2/1 -> Outport2/1
  PS-Simulink Converter/1 -> Sum/2
  t2ddknee/1 -> Scope2/1
  tddLF_knee/1 -> Sum/1
  connections:
  Knee joint/RConn2 -- q/RConn1 -- PS-Simulink Converter3/LConn1
  Knee joint/LConn1 -- Conn1/RConn1
  Conn2/RConn1 -- Knee joint/RConn1
  PS-Simulink Converter1/LConn1 -- Knee joint/RConn3 -- PS-Simulink Converter/LConn1
  Simulink-PS Converter/RConn1 -- Knee joint/LConn2
  PS-Simulink Converter2/LConn1 -- Knee joint/RConn4

== system final_quadruped_060722_alphaobjfun/Model/Left Leg Front /Subsystem ==
  qaa : Inport
  qhaz : Inport  Port=2
  Qquat : Inport  Port=3
  qka : Inport  Port=4
  td4 : Inport  Port=5
  td5 : Inport  Port=6
  w_torso : Inport  Port=7
  vlinks : Inport  Port=8
  v_torso : Inport  Port=9
  qhax : Inport  Port=10
  qhay : Inport  Port=11
  CMg : Inport  Port=12
  td123 : Inport  Port=13
  MATLAB Function : MATLAB Function  TreatAsAtomicUnit=on
  MATLAB Function1 : MATLAB Function  TreatAsAtomicUnit=on
  MATLAB Function2 : MATLAB Function  TreatAsAtomicUnit=on
  MATLAB Function4 : MATLAB Function  TreatAsAtomicUnit=on
  To Workspace : ToWorkspace  VariableName=h_dotLF  SaveFormat=Timeseries  SampleTime=-1
  To Workspace2 : ToWorkspace  VariableName=eb4g  SaveFormat=Timeseries  SampleTime=-1
  To Workspace4 : ToWorkspace  VariableName=eb5g  SaveFormat=Timeseries  SampleTime=-1
  To Workspace5 : ToWorkspace  VariableName=cmb4  SaveFormat=Timeseries  SampleTime=-1
  To Workspace6 : ToWorkspace  VariableName=ab3g  SaveFormat=Timeseries  SampleTime=-1
  To Workspace7 : ToWorkspace  VariableName=ab4g  SaveFormat=Timeseries  SampleTime=-1
  To Workspace8 : ToWorkspace  VariableName=cmb5  SaveFormat=Timeseries  SampleTime=-1
  hLF : Outport
  h_dotLF : Outport  Port=2
  Qd5g : Outport  Port=3
  alpLF : Outport  Port=4
  wires:
  MATLAB Function/12(cmb3g) -> MATLAB Function1/9(cmb3)
  MATLAB Function/8(ab3g) -> MATLAB Function4/6(ab4g), To Workspace6/1, MATLAB Function1/7(ab30g)
  MATLAB Function/9(ab4g) -> MATLAB Function1/12(ab40g), To Workspace7/1, MATLAB Function4/7(eb5g)
  MATLAB Function/4(eb4g) -> MATLAB Function2/7(eb4g), To Workspace2/1, MATLAB Function1/4(eb40g), MATLAB Function4/4(eb4g)
  MATLAB Function/14(cmb5g) -> To Workspace8/1, MATLAB Function1/10(cmb5)
  MATLAB Function/3(eb3g) -> MATLAB Function2/6(eb3g), MATLAB Function4/3(eb3g), MATLAB Function1/3(eb30g)
  MATLAB Function/13(cmb4g) -> MATLAB Function1/8(cmb4), To Workspace5/1
  MATLAB Function/5(eb5g) -> MATLAB Function2/8(eb5g), MATLAB Function4/5(ab3g), To Workspace4/1, MATLAB Function1/11(eb50g)
  MATLAB Function1/1(hLF) -> hLF/1
  qka/1 -> MATLAB Function/6(qkb)
  qaa/1 -> MATLAB Function/4(qab)
  Qquat/1 -> MATLAB Function/5(Qquat)
  qhaz/1 -> MATLAB Function/1(qhbz)
  td123/1 -> MATLAB Function4/10(td123)
  td4/1 -> MATLAB Function4/12(td4)
  td5/1 -> MATLAB Function4/13(td5)
  vlinks/1 -> MATLAB Function4/8(vlinks)
  v_torso/1 -> MATLAB Function4/11(v_torso)
  MATLAB Function1/2(rhoLF) -> MATLAB Function2/12(rhoLF)
  MATLAB Function2/1(h_dotLF) -> To Workspace/1, h_dotLF/1
  MATLAB Function/15(Qd5g) -> Qd5g/1
  w_torso/1 -> MATLAB Function4/9(w_torso)
  qhax/1 -> MATLAB Function/2(qhbx)
  qhay/1 -> MATLAB Function/3(qhby)
  MATLAB Function/1(eb1g) -> MATLAB Function1/1(eb10g), MATLAB Function4/1(eb1g), MATLAB Function2/1(eb1g)
  MATLAB Function/2(eb2g) -> MATLAB Function2/2(eb2g), MATLAB Function4/2(eb2g), MATLAB Function1/2(eb20g)
  MATLAB Function/6(ab1g) -> MATLAB Function1/5(ab10g)
  MATLAB Function/7(ab2g) -> MATLAB Function1/6(ab20g)
  MATLAB Function/10(cmb1g) -> MATLAB Function1/13(cmb1)
  MATLAB Function/11(cmb2g) -> MATLAB Function1/14(cmb2)
  MATLAB Function4/1(eb_dg1) -> MATLAB Function2/3(eb_dg1)
  MATLAB Function4/2(eb_dg2) -> MATLAB Function2/4(eb_dg2)
  MATLAB Function4/3(eb_dg3) -> MATLAB Function2/5(eb_dg3)
  MATLAB Function4/4(eb_dg4) -> MATLAB Function2/9(eb_dg4)
  MATLAB Function4/5(eb_dg5) -> MATLAB Function2/10(eb_dg5)
  MATLAB Function4/6(rho_dotLF) -> MATLAB Function2/11(rho_dotLF)
  MATLAB Function/16(I1) -> MATLAB Function1/15(I1)
  MATLAB Function/17(I2) -> MATLAB Function1/16(I2)
  MATLAB Function/18(I3) -> MATLAB Function1/17(I3)
  MATLAB Function/19(I4) -> MATLAB Function1/18(I4)
  MATLAB Function/20(I5) -> MATLAB Function1/19(I5)
  CMg/1 -> MATLAB Function1/20(CMg)
  MATLAB Function1/3(alpLF) -> alpLF/1

== system final_quadruped_060722_alphaobjfun/Model/Right Leg Back/Ankle  ==
  note: accelerationRFankle
  tddRB_ankle : Inport
  t2ddankle : Inport  Port=2
  Ankle : sm_lib/Joints/Revolute Joint  JointMode=Normal  SenseConstraintForce=off  SenseConstraintForceX=off  SenseConstraintForceY=off  SenseConstraintForceZ=off  SenseConstraintTorque=off  SenseConstraintTorqueX=off  SenseConstraintTorqueY=off  SenseConstraintTorqueZ=off  SenseTotalForce=off  SenseTotalForceX=off  SenseTotalForceY=off  SenseTotalForceZ=off  SenseTotalTorque=off  SenseTotalTorqueX=off  SenseTotalTorqueY=off  SenseTotalTorqueZ=off  CompositeWrenchDir=FollowerOnBase  CompositeWrenchFrame=BaseFrame  EquilibriumPosition=0  EquilibriumPositionUnits=deg  SpringStiffness=0  SpringStiffnessUnits=N*m/deg  DampingCoefficient=0  DampingCoefficientUnits=N*m/(deg/s)  TorqueActuationMode=InputTorque  MotionActuationMode=ComputedMotion  SensePosition=on  SenseVelocity=on  SenseAcceleration=on  SenseTorqueForce=off  SenseLowerLimitTorqueForce=off  SenseUpperLimitTorqueForce=off  LowerLimitSpecify=off  LowerLimitBound=-90  LowerLimitBoundUnits=deg  LowerLimitStiffness=1e4  LowerLimitStiffnessUnits=N*m/deg  LowerLimitDamping=10  LowerLimitDampingUnits=N*m/(deg/s)  LowerLimitTransitionRegionWidth=0.1  LowerLimitTransitionRegionWidthUnits=deg  UpperLimitSpecify=off  UpperLimitBound=90  UpperLimitBoundUnits=deg  UpperLimitStiffness=1e4  UpperLimitStiffnessUnits=N*m/deg  UpperLimitDamping=10  UpperLimitDampingUnits=N*m/(deg/s)  UpperLimitTransitionRegionWidth=0.1  UpperLimitTransitionRegionWidthUnits=deg  PositionTargetSpecify=on  PositionTargetPriority=Low  PositionTargetValue=-15  PositionTargetValueUnits=deg  VelocityTargetSpecify=on  VelocityTargetPriority=Low  VelocityTargetValue=1  VelocityTargetValueUnits=deg/s
  Bus Creator : BusCreator  Inputs=3
  PID Controller : pid_lib/PID Controller  Controller=PID  Form=Parallel  TimeDomain=Continuous-time  UseExternalTs=off  SampleTime=-1  IntegratorMethod=Forward Euler  FilterMethod=Forward Euler  ControllerParametersSource=internal  P=kp_ankle  I=ki_ankle  D=kd_ankle  UseFilter=on  N=100  TunerSelectOption=Transfer Function Based (PID Tuner App)  InitialConditionSource=internal  InitialConditionForIntegrator=0  InitialConditionForFilter=0  DifferentiatorICPrevScaledInput=0  ExternalReset=none  TrackingMode=off  Kt=1  LimitOutput=off  SatLimitsSource=internal  UpperSaturationLimit=inf  LowerSaturationLimit=-inf  LinearizeAsGain=on  AntiWindupMode=none  Kb=1  POutMin=[]  POutMax=[]  IOutMin=[]  IOutMax=[]  DOutMin=[]  DOutMax=[]  NOutMin=[]  NOutMax=[]  SumOutMin=[]  SumOutMax=[]  SaturationOutMin=[]  SaturationOutMax=[]  PParamMin=[]  PParamMax=[]  IParamMin=[]  IParamMax=[]  DParamMin=[]  DParamMax=[]  NParamMin=[]  NParamMax=[]  KbParamMin=[]  KbParamMax=[]  KtParamMin=[]  KtParamMax=[]  KbOutMin=[]  KbOutMax=[]  KtOutMin=[]  KtOutMax=[]  IntegratorOutMin=[]  IntegratorOutMax=[]  FilterOutMin=[]  FilterOutMax=[]  SumI1OutMin=[]  SumI1OutMax=[]  SumI2OutMin=[]  SumI2OutMax=[]  SumI3OutMin=[]  SumI3OutMax=[]  SumI4OutMin=[]  SumI4OutMax=[]  SumDOutMin=[]  SumDOutMax=[]  DifferentiatorOutMin=[]  DifferentiatorOutMax=[]  FilterDiffOutCoefMin=[]  FilterDiffOutCoefMax=[]  ReciprocalOutMin=[]  ReciprocalOutMax=[]  SumDenOutMin=[]  SumDenOutMax=[]  SumNumOutMin=[]  SumNumOutMax=[]  DivideOutMin=[]  DivideOutMax=[]  UdiffTsProdOutMin=[]  UdiffTsProdOutMax=[]  NTsProdOutMin=[]  NTsProdOutMax=[]  UintegralTsProdOutMin=[]  UintegralTsProdOutMax=[]  UngainTsProdOutMin=[]  UngainTsProdOutMax=[]  IntegratorContinuousStateAttributes=''  IntegratorStateMustResolveToSignalObject=off  IntegratorRTWStateStorageClass=Auto  FilterContinuousStateAttributes=''  FilterStateMustResolveToSignalObject=off  FilterRTWStateStorageClass=Auto  ParallelPVariant=InternalParameters  IdealPVariant=Disabled  IVariant=InternalParameters  DVariant=InternalParameters  IntegratorVariant=Continuous  SatVariant=Disabled  AWVariant=Passthrough  PCopyVariant=Disabled  TRVariant=Disabled  FdbkBlocksVariant=Forward  IdealPFdbkVariant=Disabled  SatFdbkVariant=Disabled  DerivativeFilterVariant=ContFilter  NVariant=InternalParameters  NCopyVariant=Disabled  FilterICVariant=InternalICsFilter  IntegratorICVariant=InternalICs  ExternalResetVariant=Disabled  TRSumVariant=Passthrough  SumFdbkVariant=Disabled  SumVariant=Sum_PID  TsampFilterVariant=InternalTs  TsampNgainVariant=Passthrough  TsampIntegralVariant=Passthrough  ExternalSaturationOutDataTypeStr=Inherit: Same as second input
  PS-Simulink Converter : nesl_utility/PS-Simulink Converter  PhysicalDomain=network_engine_domain  SubClassName=ps_output  LeftPortType=input  RightPortType=output  PseudoPeriodic=off  Frequencies=[]  Unit=1  AffineConversion=off
      settings: SourceProductBaseCode=PW,SS
  PS-Simulink Converter1 : nesl_utility/PS-Simulink Converter  PhysicalDomain=network_engine_domain  SubClassName=ps_output  LeftPortType=input  RightPortType=output  PseudoPeriodic=off  Frequencies=[]  Unit=1  AffineConversion=off
      settings: SourceProductBaseCode=PW,SS
  PS-Simulink Converter2 : nesl_utility/PS-Simulink Converter  PhysicalDomain=network_engine_domain  SubClassName=ps_output  LeftPortType=input  RightPortType=output  PseudoPeriodic=off  Frequencies=[]  Unit=inherit  AffineConversion=off
      settings: SourceProductBaseCode=PW,SS
  PS-Simulink Converter3 : nesl_utility/PS-Simulink Converter  PhysicalDomain=network_engine_domain  SubClassName=ps_output  LeftPortType=input  RightPortType=output  PseudoPeriodic=off  Frequencies=[]  Unit=inherit  AffineConversion=off
      settings: SourceProductBaseCode=PW,SS
  PS-Simulink Converter4 : nesl_utility/PS-Simulink Converter  PhysicalDomain=network_engine_domain  SubClassName=ps_output  LeftPortType=input  RightPortType=output  PseudoPeriodic=off  Frequencies=[]  Unit=inherit  AffineConversion=off
      settings: SourceProductBaseCode=PW,SS
  Scope : Scope
  Scope1 : Scope
  Scope2 : Scope
  Simulink-PS Converter : nesl_utility/Simulink-PS Converter  PhysicalDomain=network_engine_domain  SubClassName=ps_input  LeftPortType=input  RightPortType=output  PseudoPeriodic=off  Frequencies=[]  NoiseDistribution=none  NoiseParameters=[]  Unit=1  AffineConversion=off  FilteringAndDerivatives=provide  SimscapeFilterOrder=1  InputFilterTimeConstant=0.001  UdotUserProvided=0
      settings: SourceProductBaseCode=PW,SS
  Sum : Sum  Inputs=|+-
  B : PMIOPort  Side=Left
  F : PMIOPort  Port=2  Side=Right
  meas : Outport  VectorParamsAs1DForOutWhenUnconnected=off
  Outport : Outport  Port=2
  Outport1 : Outport  Port=3
  Outport2 : Outport  Port=4
  wires:
  PS-Simulink Converter1/1 -> Bus Creator/1  "angleRFankle"
  PS-Simulink Converter/1 -> Outport1/1, Bus Creator/2  "speedRFankle"
  PID Controller/1 -> Scope1/1, Simulink-PS Converter/1, Bus Creator/3  "torqueRFankle"
  Bus Creator/1 -> meas/1
  Sum/1 -> PID Controller/1, Scope/1
  PS-Simulink Converter2/1 -> Outport/1
  PS-Simulink Converter3/1 -> Outport2/1
  PS-Simulink Converter4/1 -> Sum/2
  tddRB_ankle/1 -> Sum/1
  t2ddankle/1 -> Scope2/1
  connections:
  F/RConn1 -- Ankle/RConn1
  Ankle/LConn1 -- B/RConn1
  PS-Simulink Converter1/LConn1 -- Ankle/RConn2 -- PS-Simulink Converter2/LConn1
  Ankle/RConn3 -- PS-Simulink Converter4/LConn1 -- PS-Simulink Converter/LConn1
  Simulink-PS Converter/RConn1 -- Ankle/LConn2
  Ankle/RConn4 -- PS-Simulink Converter3/LConn1
